simulink model "n_i_loop"  (R2015b)
settings: Solver=ode45  StartTime=0.0  StopTime=2  RelTol=1e-3
settings Model: Creator=Administrator  LastModifiedBy=Administrator

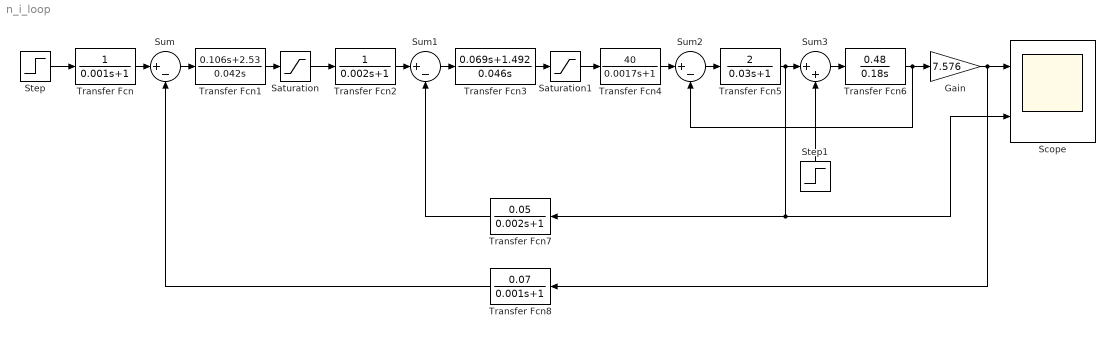
== system n_i_loop ==
  Gain : Gain  Gain=7.576
  Saturation : Saturate  UpperLimit=8  LowerLimit=-8
  Saturation1 : Saturate  UpperLimit=5  LowerLimit=-5
  Scope : Scope  NumInputPorts=2
  Step : Step  Time=0  After=150  SampleTime=0
  Step1 : Step  Time=0  After=0  SampleTime=0
  Sum : Sum  Inputs=|+-
  Sum1 : Sum  Inputs=|+-
  Sum2 : Sum  Inputs=|+-
  Sum3 : Sum  Inputs=|++
  Transfer Fcn : TransferFcn  Denominator=[0.001 1]
  Transfer Fcn1 : TransferFcn  Numerator=[0.106 2.53]  Denominator=[0.042 0]
  Transfer Fcn2 : TransferFcn  Denominator=[0.002 1]
  Transfer Fcn3 : TransferFcn  Numerator=[0.069 1.492]  Denominator=[0.046 0]
  Transfer Fcn4 : TransferFcn  Numerator=[40]  Denominator=[0.0017 1]
  Transfer Fcn5 : TransferFcn  Numerator=[2]  Denominator=[0.03 1]
  Transfer Fcn6 : TransferFcn  Numerator=[0.48]  Denominator=[0.18 0]
  Transfer Fcn7 : TransferFcn  Numerator=[0.05]  Denominator=[0.002 1]
  Transfer Fcn8 : TransferFcn  Numerator=[0.07]  Denominator=[0.001 1]
  wires:
  Transfer Fcn/1 -> Sum/1
  Step/1 -> Transfer Fcn/1
  Sum/1 -> Transfer Fcn1/1
  Transfer Fcn1/1 -> Saturation/1
  Saturation/1 -> Transfer Fcn2/1
  Transfer Fcn2/1 -> Sum1/1
  Sum1/1 -> Transfer Fcn3/1
  Transfer Fcn3/1 -> Saturation1/1
  Transfer Fcn4/1 -> Sum2/1
  Sum2/1 -> Transfer Fcn5/1
  Transfer Fcn5/1 -> Scope/2, Transfer Fcn7/1, Sum3/1
  Sum3/1 -> Transfer Fcn6/1
  Transfer Fcn6/1 -> Gain/1, Sum2/2
  Step1/1 -> Sum3/2
  Transfer Fcn7/1 -> Sum1/2
  Transfer Fcn8/1 -> Sum/2
  Gain/1 -> Scope/1, Transfer Fcn8/1
  Saturation1/1 -> Transfer Fcn4/1
